simulink model "week2_p1"  (R2020b)
settings: Solver=VariableStepAuto  StartTime=0.0  StopTime=10.0  RelTol=1e-3
model workspace (MAT data in the model file):
  data = 0
settings Model: Creator=admin  LastModifiedBy=admin

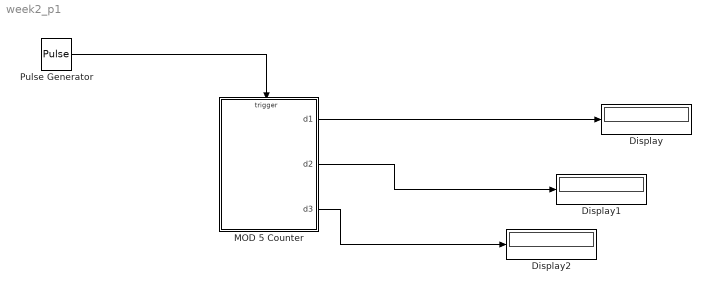
== system week2_p1 ==
  Display : Display
  Display1 : Display
  Display2 : Display
  MOD 5 Counter : Stateflow chart  TreatAsAtomicUnit=on
  Pulse Generator : DiscretePulseGenerator  PulseType=Time based  Period=10  PulseWidth=5
  wires:
  Pulse Generator/1 -> MOD 5 Counter/Trigger
  MOD 5 Counter/1(d1) -> Display/1
  MOD 5 Counter/2(d2) -> Display1/1
  MOD 5 Counter/3(d3) -> Display2/1

== stateflow chart week2_p1/MOD 5 Counter ==
  settings: executeAtInitialization=1
  state state1
    state one
      en:
      d2= 1;
    note: inputc1
    state zero
      en:
      d1 = 0;
    state two
      en:
      d1 =2;
    state four
      en:
      d1= 4;
    state three
      en:
      d1= 3;
    state1.one -> state1.two : inputc1
    state1.zero -> state1.one
    (default) -> state1.zero
    state1.four -> state1.zero : inputc1
    state1.two -> state1.three : inputc1
    state1.three -> state1.four : inputc1
  state state2
    state one
      en:
      d2= 1;
    note: inputc2
    state two
      en:
      d2 =2;
    state zero
      en:
      d2 = 0;
    state three
      en:
      d2 = 3;
    state four
      en:
      d2= 4;
    state2.one -> state2.two : inputc2
    state2.zero -> state2.one
    (default) -> state2.zero
    state2.two -> state2.three : inputc2
    state2.four -> state2.zero : inputc2
    state2.three -> state2.four : inputc2
  state state3
    state one
      en:
      d3 = 1;
    note: inputc3
    state zero
      en:
      d3 = 0;
    state two
      en:
      d3 =2;
    state four
      en:
      d3= 4;
    state three
      en:
      d3 = 3;
    state3.one -> state3.two : inputc3
    state5 -> state3.one
    (default) -> state5
    state3.four -> state5 : inputc3
    state3.two -> state3.three : inputc3
    state3.three -> state3.four : inputc3
  data: d1 output; d2 output; d3 output
  events: inputc2 local FUNCTION_CALL_EVENT; inputc3 local FUNCTION_CALL_EVENT; inputc1 input RISING_EDGE_EVENT
